simulink model "bandas"  (Simulink 7.9)
settings: Solver=ode45  StartTime=0.0  StopTime=1200  RelTol=1e-3
settings Model: Creator=root  LastModifiedBy=root

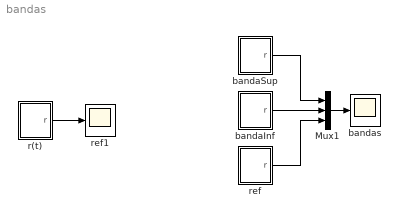
== system bandas ==
  Mux1 : Mux  Inputs=3
  bandaInf : Subsystem
  bandaSup : Subsystem
  bandas : Scope
      settings: TimeRange=971.6614906832298  YMin=14.5  YMax=22.5  SaveName=bandas
  r(t) : Subsystem
  ref : Subsystem
  ref1 : Scope
      settings: TimeRange=971.6614906832298  YMin=14.5  YMax=22.5  SaveName=referencia
  wires:
  Mux1/1 -> bandas/1
  bandaSup/1(r) -> Mux1/1
  bandaInf/1(r) -> Mux1/2
  ref/1(r) -> Mux1/3
  r(t)/1(r) -> ref1/1

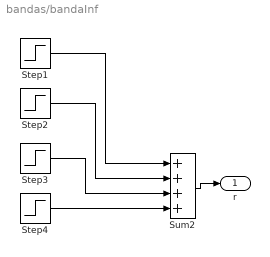
== system bandas/bandaInf ==
  Step1 : Step  Time=300  Before=22.5*0.98  After=22.5*0.98  SampleTime=0
  Step2 : Step  Time=301  After=22.5*0.98
  Step3 : Step  Time=601  After=-7.5*0.98
  Step4 : Step  Time=901  After=15*0.98
  Sum2 : Sum  Inputs=++++
  r : Outport
  wires:
  Sum2/1 -> r/1
  Step1/1 -> Sum2/1
  Step2/1 -> Sum2/2
  Step3/1 -> Sum2/3
  Step4/1 -> Sum2/4

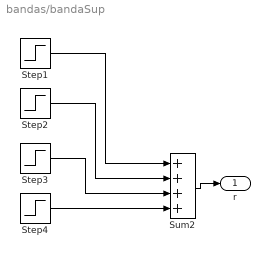
== system bandas/bandaSup ==
  Step1 : Step  Time=300  Before=22.5*(1.02)  After=22.5*(1.02)  SampleTime=0
  Step2 : Step  Time=301  After=22.5*(1.02)
  Step3 : Step  Time=601  After=-7.5*(1.02)
  Step4 : Step  Time=901  After=15*(1.02)
  Sum2 : Sum  Inputs=++++
  r : Outport
  wires:
  Sum2/1 -> r/1
  Step1/1 -> Sum2/1
  Step2/1 -> Sum2/2
  Step3/1 -> Sum2/3
  Step4/1 -> Sum2/4

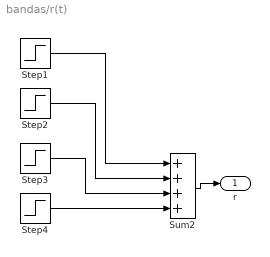
== system bandas/r(t) ==
  Step1 : Step  Time=300  Before=22.5  After=22.5  SampleTime=0
  Step2 : Step  Time=301  After=22.5
  Step3 : Step  Time=601  After=-7.5
  Step4 : Step  Time=901  After=15
  Sum2 : Sum  Inputs=++++
  r : Outport
  wires:
  Sum2/1 -> r/1
  Step1/1 -> Sum2/1
  Step2/1 -> Sum2/2
  Step3/1 -> Sum2/3
  Step4/1 -> Sum2/4

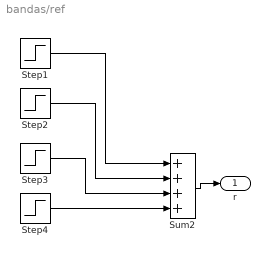
== system bandas/ref ==
  Step1 : Step  Time=300  Before=22.5  After=22.5  SampleTime=0
  Step2 : Step  Time=301  After=22.5
  Step3 : Step  Time=601  After=-7.5
  Step4 : Step  Time=901  After=15
  Sum2 : Sum  Inputs=++++
  r : Outport
  wires:
  Sum2/1 -> r/1
  Step1/1 -> Sum2/1
  Step2/1 -> Sum2/2
  Step3/1 -> Sum2/3
  Step4/1 -> Sum2/4
